simulink model "Final_Simulink_Model2020a"  (R2020a)
settings: Solver=FixedStepAuto  StartTime=0.0  StopTime=10  FixedStep=1e-3  RelTol=1e-3  EnableMultiTasking=on
undefined symbols (not defined in the file): D0, D1, D10, D11, D12, D13, D2, D3, D4, D5, D6, D7, D8, D9, PTA0, PTA1, PTA2, PTB23, PTB9, PTC16, PTC17, PTC2, PTC3, PTC4, PTD0, PTD1, PTD2, PTD3
libraries: frdmk64flib x14
settings Model: ExtModeTrigDuration=5  Creator=ryanb  LastModifiedBy=ryanb
settings OptimizationCC: EnhancedBackFolding=on  PassReuseOutputArgsAs=Individual arguments  ZeroExternalMemoryAtStartup=off  ZeroInternalMemoryAtStartup=off  MaxStackSize=64  OptimizeBlockOrder=speed  DifferentSizesBufferReuse=on  OptimizationCustomize=off  EfficientTunableParamExpr=on
settings DebuggingCC: ParameterTunabilityLossMsg=error  UnconnectedInputMsg=none  UnconnectedOutputMsg=none  UnconnectedLineMsg=none
settings HardwareCC: ProdBitPerPointer=32  ProdBitPerSizeT=32  ProdBitPerPtrDiffT=32  ProdLargestAtomicInteger=Long  ProdLargestAtomicFloat=Double  ProdWordSize=32  ProdHWDeviceType=ARM Compatible->ARM Cortex
settings ModelReferenceCC: EnableRefExpFcnMdlSchedulingChecks=off
settings SFSimCC: MATLABDynamicMemAlloc=off
settings RTWCC: SystemTargetFile=ert.tlc  HardwareBoard=NXP FRDM-K64F  TemplateMakefile=ert_default_tmf  Toolchain=GNU Tools for ARM Embedded Processors
settings CodeAppCC: ForceParamTrailComments=on  IgnoreCustomStorageClasses=off  OperatorAnnotations=on  SimulinkDataObjDesc=on  SFDataObjDesc=on  InsertBlockDesc=on
settings ERTTargetCC: ExtModeTransport=4  ExtModeMexFile=sendToCommService
settings SettingsController: UseSoCProfilerForTargets=0

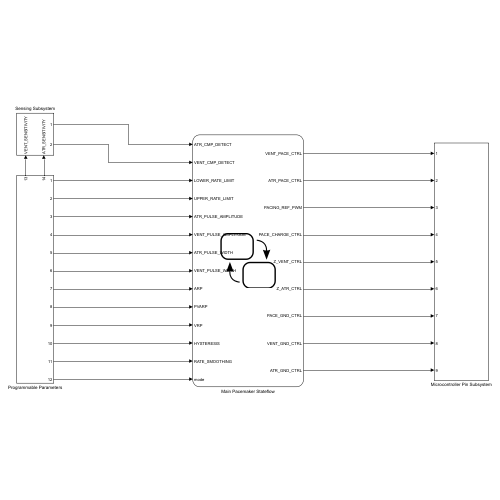
[thumbnail: Simulink's stored preview of the top-level diagram]
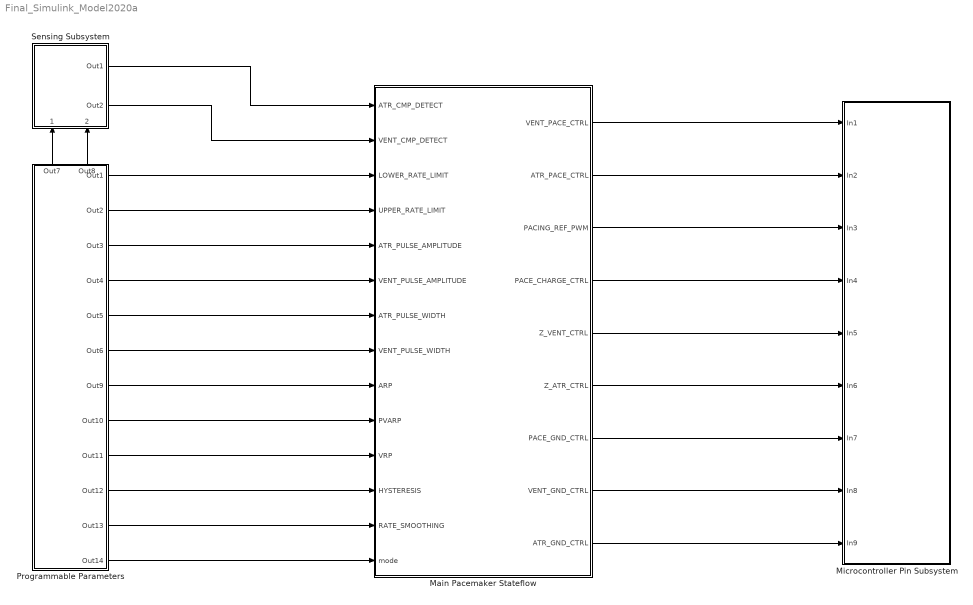
== system Final_Simulink_Model2020a ==
  Main Pacemaker Stateflow : Stateflow chart  TreatAsAtomicUnit=on
      settings: PortSchema="{\"entries\":[{\"content\":{\"sides\":[{\"content\":{\"connectorIds\":[\"In1\",\"In2\",\"In3\",\"In4\",\"In7\",\"In5\",\"In8\",\"In6\",\"In9\",\"In10\",\"In11\",\"In12\",\"In13\",\"In14\"]},\"type\":\"ConnectorPlacement.EquallySpacedRectSide\",\"uuid\":\"e04c6c9d-b568-4760-aae3-37103fc4b8a5\"},{\"content\":{\"connectorIds\":[\"Out1\",\"Out2\",\"Out3\",\"Out4\",\"Out5\",\"Out6\",\"Out7\",\"Out8\",\"Out9\"],\"side\":\"RIGHT\"},\"type\":\"ConnectorPlacement.EquallySpacedRectSide\",\"uuid\":\"410f5465-af00-4611-9887-c67099d36fd9\"},{\"content\":{\"side\":\"TOP\"},\"type\":\"ConnectorPlacement.EquallySpacedRectSide\",\"uuid\":\"117107fa-ec70-4a57-9ea7-207f77d687e8\"}]},\"type\":\"ConnectorPlacement.EquallySpacedConnector\",\"uuid\":\"376840e9-6019-4e50-8c40-c1322fd1edca\"}],\"packageUris\":[\"http://schema.mathworks.com/mf0/Connector/R2020b\"],\"version\":\"1.0\"}"
  Microcontroller Pin Subsystem : Subsystem
  Programmable Parameters : Subsystem
      settings: PortSchema="{\"entries\":[{\"content\":{\"sides\":[{\"content\":{},\"type\":\"ConnectorPlacement.EquallySpacedRectSide\",\"uuid\":\"a66c8e23-13e5-4abc-9e09-ab5de47ab8f3\"},{\"content\":{\"connectorIds\":[\"Out1\",\"Out2\",\"Out3\",\"Out4\",\"Out5\",\"Out6\",\"Out7\",\"Out8\",\"Out9\",\"Out10\",\"Out11\",\"Out12\"],\"side\":\"RIGHT\"},\"type\":\"ConnectorPlacement.EquallySpacedRectSide\",\"uuid\":\"6a9d25ad-44fc-45a2-8267-3a8c58854065\"},{\"content\":{\"connectorIds\":[\"Out13\",\"Out14\"],\"side\":\"TOP\"},\"type\":\"ConnectorPlacement.EquallySpacedRectSide\",\"uuid\":\"f44503e8-6d5f-481a-bd74-8db17b5d4837\"}]},\"type\":\"ConnectorPlacement.EquallySpacedConnector\",\"uuid\":\"c0ce9d52-7c52-4f4e-8e23-cf5f7806242f\"}],\"packageUris\":[\"http://schema.mathworks.com/mf0/Connector/R2020b\"],\"version\":\"1.0\"}"
  Sensing Subsystem : Subsystem
      settings: PortSchema="{\"entries\":[{\"content\":{\"sides\":[{\"content\":{},\"type\":\"ConnectorPlacement.EquallySpacedRectSide\",\"uuid\":\"02e0911b-3253-486a-acb8-f1ba1f788aa5\"},{\"content\":{\"connectorIds\":[\"Out1\",\"Out2\"],\"side\":\"RIGHT\"},\"type\":\"ConnectorPlacement.EquallySpacedRectSide\",\"uuid\":\"66620bda-3110-4f43-a68e-d3775ac902e4\"},{\"content\":{\"side\":\"TOP\"},\"type\":\"ConnectorPlacement.EquallySpacedRectSide\",\"uuid\":\"5a7389cd-e024-434f-a78f-666a7db32550\"},{\"content\":{\"connectorIds\":[\"In1\",\"In2\"],\"side\":\"BOTTOM\"},\"type\":\"ConnectorPlacement.EquallySpacedRectSide\",\"uuid\":\"7cfc8cd2-653b-4c46-8563-1d8a50e07e7c\"}]},\"type\":\"ConnectorPlacement.EquallySpacedConnector\",\"uuid\":\"3e76420e-71f9-4267-bc59-506d487f0d17\"}],\"packageUris\":[\"http://schema.mathworks.com/mf0/Connector/R2020b\"],\"version\":\"1.0\"}"
  wires:
  Programmable Parameters/1(Out1) -> Main Pacemaker Stateflow/3(LOWER_RATE_LIMIT)
  Programmable Parameters/2(Out2) -> Main Pacemaker Stateflow/4(UPPER_RATE_LIMIT)
  Programmable Parameters/3(Out3) -> Main Pacemaker Stateflow/7(ATR_PULSE_AMPLITUDE)
  Programmable Parameters/4(Out4) -> Main Pacemaker Stateflow/5(VENT_PULSE_AMPLITUDE)
  Programmable Parameters/5(Out5) -> Main Pacemaker Stateflow/8(ATR_PULSE_WIDTH)
  Programmable Parameters/6(Out6) -> Main Pacemaker Stateflow/6(VENT_PULSE_WIDTH)
  Programmable Parameters/13(Out7) -> Sensing Subsystem/1(VENT_SENSITIVITY)
  Programmable Parameters/14(Out8) -> Sensing Subsystem/2(ATR_SENSITIVITY)
  Programmable Parameters/7(Out9) -> Main Pacemaker Stateflow/9(ARP)
  Programmable Parameters/8(Out10) -> Main Pacemaker Stateflow/10(PVARP)
  Programmable Parameters/9(Out11) -> Main Pacemaker Stateflow/11(VRP)
  Programmable Parameters/10(Out12) -> Main Pacemaker Stateflow/12(HYSTERESIS)
  Programmable Parameters/11(Out13) -> Main Pacemaker Stateflow/13(RATE_SMOOTHING)
  Sensing Subsystem/1(Out1) -> Main Pacemaker Stateflow/1(ATR_CMP_DETECT)
  Sensing Subsystem/2(Out2) -> Main Pacemaker Stateflow/2(VENT_CMP_DETECT)
  Main Pacemaker Stateflow/1(VENT_PACE_CTRL) -> Microcontroller Pin Subsystem/1(In1)
  Main Pacemaker Stateflow/2(ATR_PACE_CTRL) -> Microcontroller Pin Subsystem/2(In2)
  Main Pacemaker Stateflow/3(PACING_REF_PWM) -> Microcontroller Pin Subsystem/3(In3)
  Main Pacemaker Stateflow/4(PACE_CHARGE_CTRL) -> Microcontroller Pin Subsystem/4(In4)
  Main Pacemaker Stateflow/5(Z_VENT_CTRL) -> Microcontroller Pin Subsystem/5(In5)
  Main Pacemaker Stateflow/6(Z_ATR_CTRL) -> Microcontroller Pin Subsystem/6(In6)
  Main Pacemaker Stateflow/7(PACE_GND_CTRL) -> Microcontroller Pin Subsystem/7(In7)
  Main Pacemaker Stateflow/8(VENT_GND_CTRL) -> Microcontroller Pin Subsystem/8(In8)
  Main Pacemaker Stateflow/9(ATR_GND_CTRL) -> Microcontroller Pin Subsystem/9(In9)
  Programmable Parameters/12(Out14) -> Main Pacemaker Stateflow/14(mode)

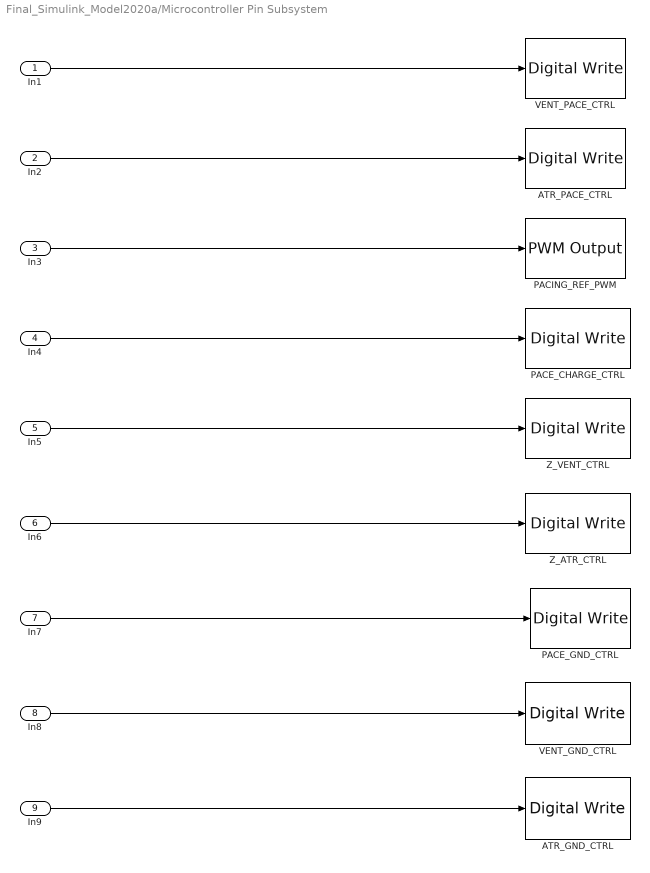
== system Final_Simulink_Model2020a/Microcontroller Pin Subsystem ==
  In1 : Inport
  In2 : Inport  Port=2
  In3 : Inport  Port=3
  In4 : Inport  Port=4
  In5 : Inport  Port=5
  In6 : Inport  Port=6
  In7 : Inport  Port=7
  In8 : Inport  Port=8
  In9 : Inport  Port=9
  ATR_GND_CTRL : frdmk64flib/Digital Write  Whichpin=PTD2 (D11)
  ATR_PACE_CTRL : frdmk64flib/Digital Write  Whichpin=PTA0 (D8)
  PACE_CHARGE_CTRL : frdmk64flib/Digital Write  Whichpin=PTB9 (D2)
  PACE_GND_CTRL : frdmk64flib/Digital Write  Whichpin=PTD0 (D10)
  PACING_REF_PWM : frdmk64flib/PWM Output  Whichpin=PTA2 (D5)  InitialFrequency=2000  InitialDutyCycle=0
  VENT_GND_CTRL : frdmk64flib/Digital Write  Whichpin=PTD3 (D12)
  VENT_PACE_CTRL : frdmk64flib/Digital Write  Whichpin=PTC4 (D9)
  Z_ATR_CTRL : frdmk64flib/Digital Write  Whichpin=PTB23 (D4)
  Z_VENT_CTRL : frdmk64flib/Digital Write  Whichpin=PTC3 (D7)
  wires:
  In5/1 -> Z_VENT_CTRL/1
  In2/1 -> ATR_PACE_CTRL/1
  In6/1 -> Z_ATR_CTRL/1
  In8/1 -> VENT_GND_CTRL/1
  In4/1 -> PACE_CHARGE_CTRL/1
  In7/1 -> PACE_GND_CTRL/1
  In3/1 -> PACING_REF_PWM/1
  In1/1 -> VENT_PACE_CTRL/1
  In9/1 -> ATR_GND_CTRL/1

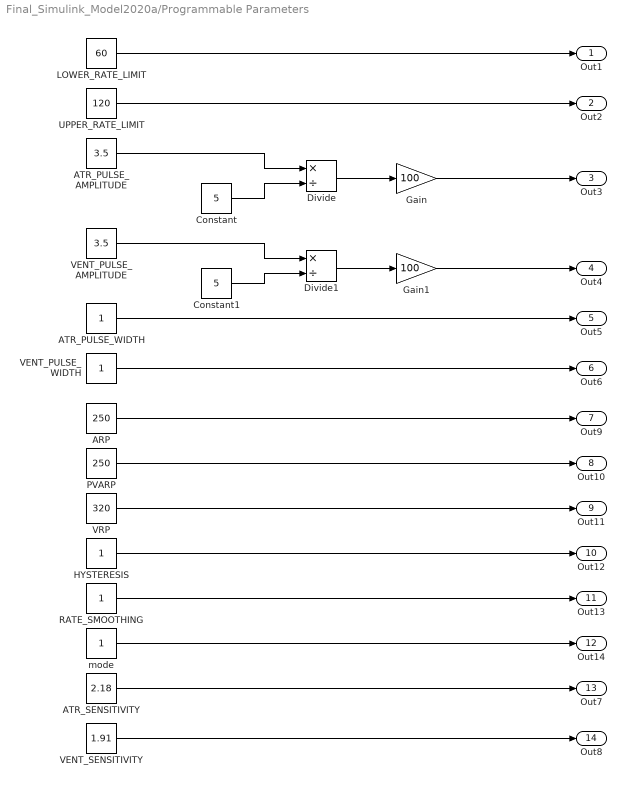
== system Final_Simulink_Model2020a/Programmable Parameters ==
  ARP : Constant  Value=250
  ATR_PULSE_AMPLITUDE : Constant  Value=3.5
  ATR_PULSE_WIDTH : Constant
  ATR_SENSITIVITY : Constant  Value=2.18
  Constant : Constant  Value=5
  Constant1 : Constant  Value=5
  Divide : Product  Inputs=*/
  Divide1 : Product  Inputs=*/
  Gain : Gain  Gain=100
  Gain1 : Gain  Gain=100
  HYSTERESIS : Constant
  LOWER_RATE_LIMIT : Constant  Value=60
  PVARP : Constant  Value=250
  RATE_SMOOTHING : Constant
  UPPER_RATE_LIMIT : Constant  Value=120
  VENT_PULSE_AMPLITUDE : Constant  Value=3.5
  VENT_PULSE_WIDTH : Constant
  VENT_SENSITIVITY : Constant  Value=1.91
  VRP : Constant  Value=320
  mode : Constant
  Out1 : Outport
  Out2 : Outport  Port=2
  Out3 : Outport  Port=3
  Out4 : Outport  Port=4
  Out5 : Outport  Port=5
  Out6 : Outport  Port=6
  Out9 : Outport  Port=7
  Out10 : Outport  Port=8
  Out11 : Outport  Port=9
  Out12 : Outport  Port=10
  Out13 : Outport  Port=11
  Out14 : Outport  Port=12
  Out7 : Outport  Port=13
  Out8 : Outport  Port=14
  wires:
  VENT_SENSITIVITY/1 -> Out8/1
  PVARP/1 -> Out10/1
  HYSTERESIS/1 -> Out12/1
  ATR_SENSITIVITY/1 -> Out7/1
  ARP/1 -> Out9/1
  VRP/1 -> Out11/1
  RATE_SMOOTHING/1 -> Out13/1
  UPPER_RATE_LIMIT/1 -> Out2/1
  LOWER_RATE_LIMIT/1 -> Out1/1
  ATR_PULSE_AMPLITUDE/1 -> Divide/1
  Constant/1 -> Divide/2
  VENT_PULSE_AMPLITUDE/1 -> Divide1/1
  Constant1/1 -> Divide1/2
  Gain/1 -> Out3/1
  Divide/1 -> Gain/1
  Divide1/1 -> Gain1/1
  Gain1/1 -> Out4/1
  ATR_PULSE_WIDTH/1 -> Out5/1
  VENT_PULSE_WIDTH/1 -> Out6/1
  mode/1 -> Out14/1

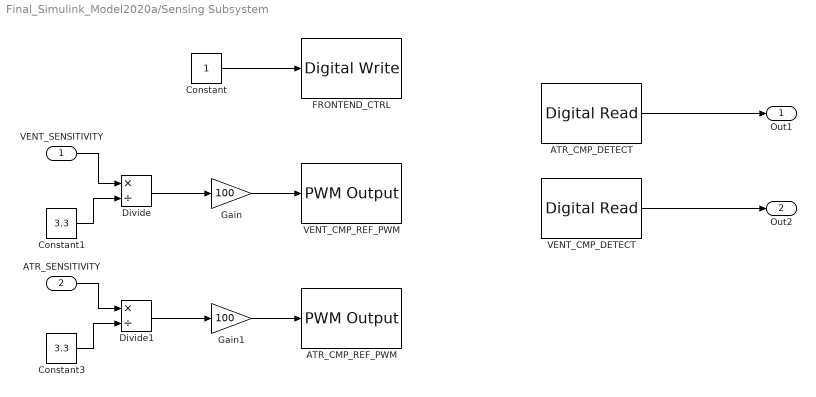
== system Final_Simulink_Model2020a/Sensing Subsystem ==
  VENT_SENSITIVITY : Inport
  ATR_SENSITIVITY : Inport  Port=2
  ATR_CMP_DETECT : frdmk64flib/Digital Read  Whichpin=PTC16 (D0)  SampleTime=-1
  ATR_CMP_REF_PWM : frdmk64flib/PWM Output  Whichpin=PTC2 (D6)  InitialFrequency=2000  InitialDutyCycle=0
  Constant : Constant
  Constant1 : Constant  Value=3.3
  Constant3 : Constant  Value=3.3
  Divide : Product  Inputs=*/
  Divide1 : Product  Inputs=*/
  FRONTEND_CTRL : frdmk64flib/Digital Write  Whichpin=PTD1 (D13)
  Gain : Gain  Gain=100
  Gain1 : Gain  Gain=100
  VENT_CMP_DETECT : frdmk64flib/Digital Read  Whichpin=PTC17 (D1)  SampleTime=-1
  VENT_CMP_REF_PWM : frdmk64flib/PWM Output  Whichpin=PTA1 (D3)  InitialFrequency=2000  InitialDutyCycle=0
  Out1 : Outport
  Out2 : Outport  Port=2
  wires:
  VENT_CMP_DETECT/1 -> Out2/1
  ATR_CMP_DETECT/1 -> Out1/1
  VENT_SENSITIVITY/1 -> Divide/1
  Constant1/1 -> Divide/2
  Constant3/1 -> Divide1/2
  ATR_SENSITIVITY/1 -> Divide1/1
  Gain1/1 -> ATR_CMP_REF_PWM/1
  Gain/1 -> VENT_CMP_REF_PWM/1
  Divide/1 -> Gain/1
  Divide1/1 -> Gain1/1
  Constant/1 -> FRONTEND_CTRL/1

== stateflow chart Final_Simulink_Model2020a/Main Pacemaker Stateflow ==
  state Startup
  state VOO
    state PACING
      entry:
      PACE_CHARGE_CTRL = 0;
      PACE_GND_CTRL = 1;
      ATR_PACE_CTRL = 0;
      ATR_GND_CTRL = 0;
      Z_ATR_CTRL = 0;
      Z_VENT_CTRL = 0;
      VENT_GND_CTRL = 0;
      VENT_PACE_CTRL = 1;
    state CHARGING
      entry:
      %%Charging C22
      ATR_PACE_CTRL = 0;
      VENT_PACE_CTRL = 0;
      PACE_CHARGE_CTRL = 1;
      %%Discharging Blocking Cap
      PACE_GND_CTRL = 1;
      Z_ATR_CTRL = 0;
      Z_VENT_CTRL = 0;
      ATR_GND_CTRL = 0;
      VENT_GND_CTRL = 1;
      PACING_REF_PWM = VENT_PULSE_AMPLITUDE;
    VOO.CHARGING -> VOO.PACING [order 2] : %%Pace Ready
        | [after(1/(LOWER_RATE_LIMIT/60000) - VENT_PULSE_WIDTH, msec)]
    VOO.PACING -> VOO.CHARGING : %%Recharge Ready
        | [after(VENT_PULSE_WIDTH, msec)]
  state AOO
    state PACING
      entry:
      PACE_CHARGE_CTRL = 0;
      PACE_GND_CTRL = 1;
      ATR_PACE_CTRL = 1;
      ATR_GND_CTRL = 0;
      Z_ATR_CTRL = 0;
      Z_VENT_CTRL = 0;
      VENT_GND_CTRL = 0;
      VENT_PACE_CTRL = 0;
    state CHARGING
      entry:
      %%Charging C22
      ATR_PACE_CTRL = 0;
      VENT_PACE_CTRL = 0;
      PACE_CHARGE_CTRL = 1;
      %%Discharging Blocking Cap
      PACE_GND_CTRL = 1;
      Z_ATR_CTRL = 0;
      Z_VENT_CTRL = 0;
      ATR_GND_CTRL = 1;
      VENT_GND_CTRL = 0;
      PACING_REF_PWM = ATR_PULSE_AMPLITUDE;
    AOO.CHARGING -> AOO.PACING [order 1] : %%Pace Ready
        | [after(1/(LOWER_RATE_LIMIT/60000) - ATR_PULSE_WIDTH, msec)]
    AOO.PACING -> AOO.CHARGING : %%Recharge Ready
        | [after(ATR_PULSE_WIDTH, msec)]
  state VVI
    state CHARGING
      entry:
      %%Charging C22
      ATR_PACE_CTRL = 0;
      VENT_PACE_CTRL = 0;
      PACE_CHARGE_CTRL = 1;
      %%Discharging Blocking Cap
      PACE_GND_CTRL = 1;
      Z_ATR_CTRL = 0;
      Z_VENT_CTRL = 0;
      ATR_GND_CTRL = 0;
      VENT_GND_CTRL = 1;
      PACING_REF_PWM = VENT_PULSE_AMPLITUDE;
    state PACING
      entry:
      PACE_CHARGE_CTRL = 0;
      PACE_GND_CTRL = 1;
      ATR_PACE_CTRL = 0;
      ATR_GND_CTRL = 0;
      Z_ATR_CTRL = 0;
      Z_VENT_CTRL = 0;
      VENT_GND_CTRL = 0;
      VENT_PACE_CTRL = 1;
    (junction 128) -> VVI.PACING [order 1] : %%Pace Ready
        | [after(1/(LOWER_RATE_LIMIT/60000) - VENT_PULSE_WIDTH - VRP, msec) && VENT_CMP_DETECT == false]
    VVI.CHARGING -> (junction 128) [order 1] : [after(VRP, msec)]
    (junction 128) -> VVI.CHARGING [order 2] : [VENT_CMP_DETECT == true]
    VVI.PACING -> VVI.CHARGING : [after(VENT_PULSE_WIDTH, msec)]
  state AAI
    state PACING
      entry:
      PACE_CHARGE_CTRL = 0;
      PACE_GND_CTRL = 1;
      ATR_PACE_CTRL = 1;
      ATR_GND_CTRL = 0;
      Z_ATR_CTRL = 0;
      Z_VENT_CTRL = 0;
      VENT_GND_CTRL = 0;
      VENT_PACE_CTRL = 0;
    state CHARGING
      entry:
      %%Charging C22
      ATR_PACE_CTRL = 0;
      VENT_PACE_CTRL = 0;
      PACE_CHARGE_CTRL = 1;
      %%Discharging Blocking Cap
      PACE_GND_CTRL = 1;
      Z_ATR_CTRL = 0;
      Z_VENT_CTRL = 0;
      ATR_GND_CTRL = 1;
      VENT_GND_CTRL = 0;
      PACING_REF_PWM = ATR_PULSE_AMPLITUDE;
    (junction 142) -> AAI.PACING [order 1] : %%Pace Ready
        | [after(1/(LOWER_RATE_LIMIT/60000) - ATR_PULSE_WIDTH - ARP, msec) && ATR_CMP_DETECT == false]
    AAI.CHARGING -> (junction 142) [order 1] : [after(ARP, msec)]
    (junction 142) -> AAI.CHARGING [order 2] : [ATR_CMP_DETECT == true]
    AAI.PACING -> AAI.CHARGING : %%Recharge Ready
        | [after(ATR_PULSE_WIDTH, msec)]
  AAI.CHARGING -> Startup [order 2] : [mode ~= 4]
  AOO.CHARGING -> Startup [order 2] : [mode ~= 2]
  VVI.CHARGING -> Startup [order 2] : [mode ~= 3]
  Startup -> VOO.CHARGING [order 3] : [mode == 1]
  VOO.CHARGING -> Startup [order 1] : [mode ~= 1]
  (default) -> Startup
  Startup -> AOO.CHARGING [order 1] : [mode == 2]
  Startup -> VVI.CHARGING [order 2] : [mode == 3]
  Startup -> AAI.CHARGING [order 4] : [mode == 4]
  data: ATR_CMP_DETECT input; VENT_CMP_DETECT input; VENT_PACE_CTRL output; ATR_PACE_CTRL output; PACING_REF_PWM output; PACE_CHARGE_CTRL output; Z_VENT_CTRL output; Z_ATR_CTRL output; PACE_GND_CTRL output; VENT_GND_CTRL output; ATR_GND_CTRL output; LOWER_RATE_LIMIT input; UPPER_RATE_LIMIT input; VENT_PULSE_AMPLITUDE input; VENT_PULSE_WIDTH input; ATR_PULSE_AMPLITUDE input; ATR_PULSE_WIDTH input; ARP input; PVARP input; VRP input; HYSTERESIS input; RATE_SMOOTHING input; mode input
